simulink model "Copter_System_discrete"  (Simulink 7.4)
settings: Solver=ode4  StartTime=0.0  StopTime=tend  FixedStep=Ts  RelTol=1e-3
values from neighbouring files (symbols this model uses):
  dis_thrust = round(thrust.*shift)    [quadrocopter_param.m]
  f1 = (I_y-I_z)/I_x    [quadrocopter_param.m]
  f2 = rot.J_z/I_x    [quadrocopter_param.m]
  f3 = (I_z-I_x)/I_y    [quadrocopter_param.m]
  f4 = rot.J_z/I_y    [quadrocopter_param.m]
  g = 9.81    [complementary_filter_param.m]    (also in quadrocopter_param.m)
  HPF = 0.95    [complementary_filter_param.m]    (also in quadrocopter_param.m)
  I_x = elec.I_x+bat.I_x+2*boom.I_1x+2*boom.I_1y+2*mot.I_1x+2*mot.I_1y+                             2*rot.I_1x+2*rot.I_1y    [quadrocopter_param.m]
  I_y = elec.I_y+bat.I_y+2*boom.I_1x+2*boom.I_1y+2*mot.I_1x+2*mot.I_1y+                             2*rot.I_1x+2*rot.I_1y    [quadrocopter_param.m]
  I_z = elec.I_z+bat.I_z+4*boom.I_1z+4*mot.I_1z+4*rot.I_1z    [quadrocopter_param.m]
  LPF = 0.05    [complementary_filter_param.m]    (also in quadrocopter_param.m)
  m = elec.m+bat.m+boom.m+(4*mot.m)+(4*rot.m)    [quadrocopter_param.m]
  rpm = [1988 2544 2940 3566 4033 4500 5033 5233]    [quadrocopter_param.m]
  shift = 1000    [quadrocopter_param.m]
  speed = rpm.*(2*pi/60)    [quadrocopter_param.m]
  thrust = [0.58 1 1.33 2 2.54 3.33 4.08 4.54]    [quadrocopter_param.m]
  Ts = 0.01    [complementary_filter_param.m]    (also in quadrocopter_param.m)
undefined symbols (not defined in the file or in its folder): boom, DiscIntNeverNeededParam
libraries: simulink x11, dspinverses x1
settings Model: Creator=Joachim  LastModifiedBy=Sreekanth
settings DataIOCC: LimitDataPoints=off  SaveOutput=off  SaveState=on

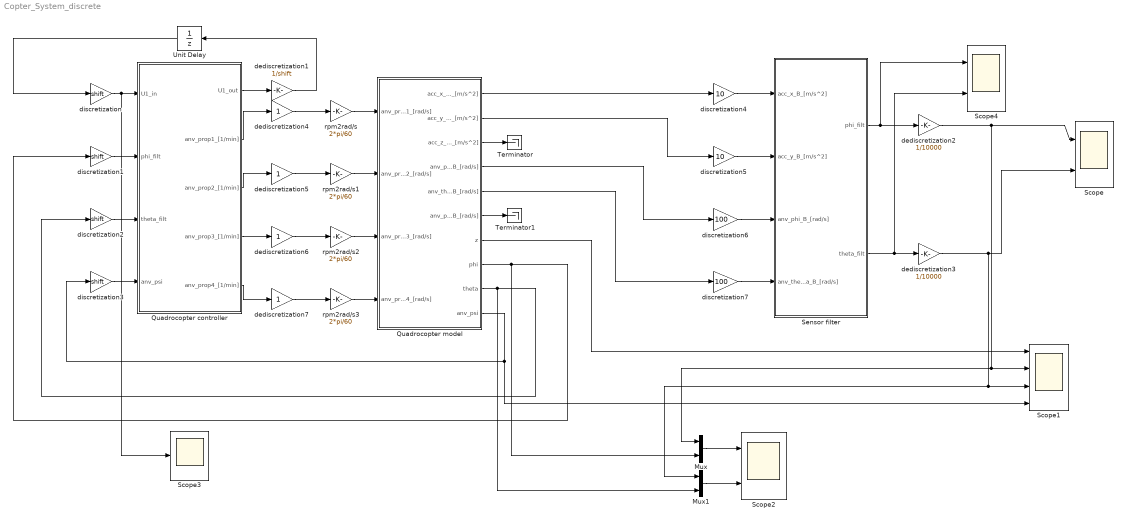
== system Copter_System_discrete ==
  Mux : Mux  Inputs=2
  Mux1 : Mux  Inputs=2
  Quadrocopter controller : Subsystem
  Quadrocopter model : Subsystem
  Scope : Scope  NumInputPorts=2
      settings: YMin=-5~-5  YMax=5~5  SaveName=ScopeData12
  Scope1 : Scope  NumInputPorts=4
      settings: YMin=-5~-5~-5~-5  YMax=5~5~5~5  SaveName=ScopeData14
  Scope2 : Scope  NumInputPorts=2
      settings: TimeRange=2.768662838392125  YMin=-0.00272445~-0.0178576  YMax=0.0152582~0.00343767  SaveName=ScopeData15
  Scope3 : Scope
      settings: TimeRange=2.768662838392125  YMin=-0.00272445  YMax=0.0152582  SaveName=ScopeData25
  Scope4 : Scope  NumInputPorts=2
      settings: YMin=-5~-5  YMax=5~5  SaveName=ScopeData27
  Sensor filter : Subsystem
  Terminator : Terminator
  Terminator1 : Terminator
  Unit Delay : UnitDelay  SampleTime=-1
  dediscretization1 : Gain  Gain=1/shift  ParameterDataType=fixdt(1, 16)  ParameterScaling=2^0  OutDataTypeMode=double  OutDataType=fixdt(1, 16)  OutScaling=2^0  OutDataTypeStr=double
  dediscretization2 : Gain  Gain=1/10000  ParameterDataType=fixdt(1, 16)  ParameterScaling=2^0  OutDataTypeMode=double  OutDataType=fixdt(1, 16)  OutScaling=2^0  OutDataTypeStr=double
  dediscretization3 : Gain  Gain=1/10000  ParameterDataType=fixdt(1, 16)  ParameterScaling=2^0  OutDataTypeMode=double  OutDataType=fixdt(1, 16)  OutScaling=2^0  OutDataTypeStr=double
  dediscretization{4..7} (4 alike) : Gain  ParameterDataType=fixdt(1, 16)  ParameterScaling=2^0  OutDataTypeMode=double  OutDataType=fixdt(1, 16)  OutScaling=2^0  OutDataTypeStr=double
  discretization{,1..3} (4 alike) : Gain  Gain=shift  ParameterDataType=fixdt(1, 16)  ParameterScaling=2^0  OutDataTypeMode=int16  OutDataType=fixdt(1, 16)  OutScaling=2^0  OutDataTypeStr=int16
  discretization4 : Gain  Gain=10  ParameterDataType=fixdt(1, 16)  ParameterScaling=2^0  OutDataTypeMode=int16  OutDataType=fixdt(1, 16)  OutScaling=2^0  OutDataTypeStr=int16
  discretization5 : Gain  Gain=10  ParameterDataType=fixdt(1, 16)  ParameterScaling=2^0  OutDataTypeMode=int16  OutDataType=fixdt(1, 16)  OutScaling=2^0  OutDataTypeStr=int16
  discretization6 : Gain  Gain=100  ParameterDataType=fixdt(1, 16)  ParameterScaling=2^0  OutDataTypeMode=int16  OutDataType=fixdt(1, 16)  OutScaling=2^0  OutDataTypeStr=int16
  discretization7 : Gain  Gain=100  ParameterDataType=fixdt(1, 16)  ParameterScaling=2^0  OutDataTypeMode=int16  OutDataType=fixdt(1, 16)  OutScaling=2^0  OutDataTypeStr=int16
  rpm2rad/s{,1..3} (4 alike) : Gain  Gain=2*pi/60  ParameterDataType=fixdt(1, 16)  ParameterScaling=2^0  OutDataType=fixdt(1, 16)  OutScaling=2^0
  wires:
  Quadrocopter controller/2(anv_prop1_[1/min]) -> dediscretization4/1
  Quadrocopter controller/3(anv_prop2_[1/min]) -> dediscretization5/1
  Quadrocopter controller/4(anv_prop3_[1/min]) -> dediscretization6/1
  Quadrocopter controller/5(anv_prop4_[1/min]) -> dediscretization7/1
  Quadrocopter model/7(z) -> Scope1/1
  Quadrocopter model/10(anv_psi) -> Scope1/4, discretization3/1
  Sensor filter/1(phi_filt) -> dediscretization2/1, Scope4/1
  Sensor filter/2(theta_filt) -> dediscretization3/1, Scope4/2
  Quadrocopter model/8(phi) -> Mux/2, discretization1/1
  Quadrocopter model/9(theta) -> Mux1/2, discretization2/1
  Mux/1 -> Scope2/1
  Mux1/1 -> Scope2/2
  Quadrocopter model/1(acc_x_B_[m/s^2]) -> discretization4/1
  Quadrocopter model/2(acc_y_B_[m/s^2]) -> discretization5/1
  Quadrocopter model/4(anv_phi_B_[rad/s]) -> discretization6/1
  Quadrocopter model/5(anv_theta_B_[rad/s]) -> discretization7/1
  Quadrocopter model/6(anv_psi_B_[rad/s]) -> Terminator1/1
  Quadrocopter model/3(acc_z_B_[m/s^2]) -> Terminator/1
  rpm2rad/s/1 -> Quadrocopter model/1(anv_prop1_[rad/s])
  rpm2rad/s1/1 -> Quadrocopter model/2(anv_prop2_[rad/s])
  rpm2rad/s2/1 -> Quadrocopter model/3(anv_prop3_[rad/s])
  rpm2rad/s3/1 -> Quadrocopter model/4(anv_prop4_[rad/s])
  discretization/1 -> Quadrocopter controller/1(U1_in), Scope3/1
  discretization1/1 -> Quadrocopter controller/2(phi_filt)
  discretization2/1 -> Quadrocopter controller/3(theta_filt)
  discretization3/1 -> Quadrocopter controller/4(anv_psi)
  dediscretization4/1 -> rpm2rad/s/1
  dediscretization5/1 -> rpm2rad/s1/1
  dediscretization6/1 -> rpm2rad/s2/1
  dediscretization7/1 -> rpm2rad/s3/1
  Quadrocopter controller/1(U1_out) -> dediscretization1/1
  dediscretization1/1 -> Unit Delay/1
  Unit Delay/1 -> discretization/1
  discretization4/1 -> Sensor filter/1(acc_x_B_[m/s^2])
  discretization5/1 -> Sensor filter/2(acc_y_B_[m/s^2])
  discretization6/1 -> Sensor filter/3(anv_phi_B_[rad/s])
  discretization7/1 -> Sensor filter/4(anv_theta_B_[rad/s])
  dediscretization2/1 -> Scope/1, Scope1/2, Mux/1
  dediscretization3/1 -> Scope/2, Scope1/3, Mux1/1

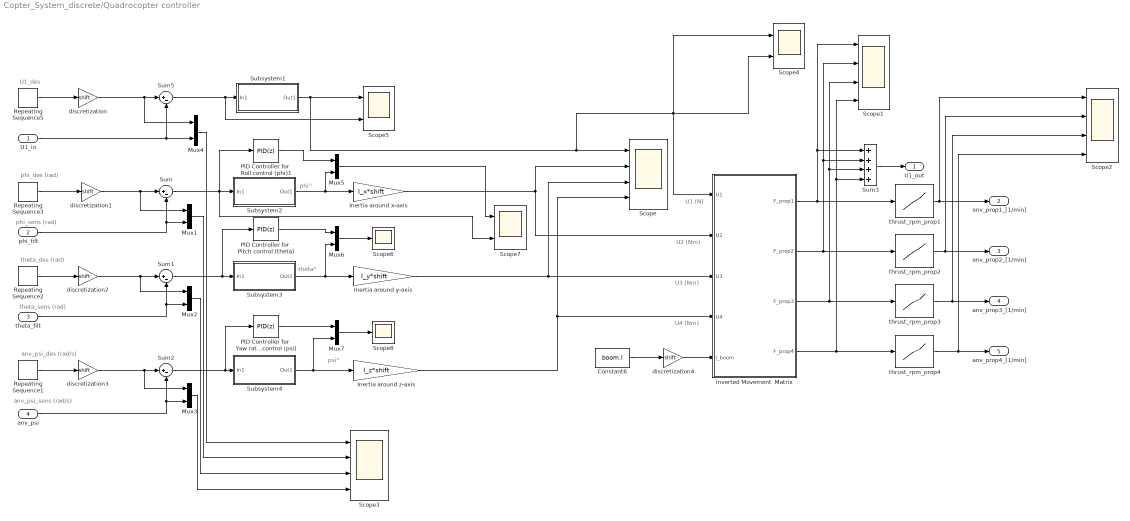
== system Copter_System_discrete/Quadrocopter controller ==
  note: U1 (N)
  note: U4 (Nm)
  note: U3 (Nm)
  note: U2 (Nm)
  note: anv_psi_sens (rad/s)
  note: anv_psi_des (rad/s)
  note: theta_sens (rad)
  note: theta_des (rad)
  note: phi_sens (rad)
  note: phi_des (rad)
  note: phi''
  note: theta''
  note: psi''
  note: U1_des
  U1_in : Inport  OutDataType=fixdt(1, 16)  OutScaling=2^0
  phi_filt : Inport  Port=2  OutDataType=fixdt(1, 16)  OutScaling=2^0
  theta_filt : Inport  Port=3  OutDataType=fixdt(1, 16)  OutScaling=2^0
  anv_psi : Inport  Port=4  OutDataType=fixdt(1, 16)  OutScaling=2^0
  Constant6 : Constant  Value=boom.l  OutDataType=fixdt(1, 16)  OutScaling=2^0  SampleTime=Ts
  Inertia around x-axis : Gain  Gain=I_x*shift  ParameterDataType=fixdt(1, 16)  ParameterScaling=2^0  OutDataType=fixdt(1, 16)  OutScaling=2^0  OutDataTypeStr=Inherit: Same as input
  Inertia around y-axis : Gain  Gain=I_y*shift  ParameterDataType=fixdt(1, 16)  ParameterScaling=2^0  OutDataType=fixdt(1, 16)  OutScaling=2^0  OutDataTypeStr=Inherit: Same as input
  Inertia around z-axis : Gain  Gain=I_z*shift  ParameterDataType=fixdt(1, 16)  ParameterScaling=2^0  OutDataType=fixdt(1, 16)  OutScaling=2^0  OutDataTypeStr=Inherit: Same as input
  Mux{1..7} (7 alike) : Mux  Inputs=2
  PID Controller for  Pitch control (theta) : simulink/Continuous/PID Controller  DialogController=pidpack.PIDConfig.pidDDGCreate  DialogControllerArgs=DataTag0  SystemSampleTime=-1  Controller=PID  TimeDomain=Discrete-time  SampleTime=Ts  IntegratorMethod=Forward Euler  FilterMethod=Forward Euler  Form=Parallel  P=20  I=5  D=10  N=100  InitialConditionSource=internal  InitialConditionForIntegrator=0  InitialConditionForFilter=0  ExternalReset=none  LimitOutput=off  UpperSaturationLimit=20  LowerSaturationLimit=-20  LinearizeAsGain=off  AntiWindupMode=clamping  Kb=1  TrackingMode=off  Kt=1  RndMeth=Nearest  PParamMin=[]  PParamMax=[]  PParamDataTypeStr=int16  IParamMin=[]  IParamMax=[]  IParamDataTypeStr=int16  DParamMin=[]  DParamMax=[]  DParamDataTypeStr=int16  NParamMin=[]  NParamMax=[]  NParamDataTypeStr=int16  KbParamMin=[]  KbParamMax=[]  KtParamMin=[]  KtParamMax=[]  POutMin=[]  POutMax=[]  POutDataTypeStr=int16  IOutMin=[]  IOutMax=[]  IOutDataTypeStr=int16  DOutMin=[]  DOutMax=[]  DOutDataTypeStr=int16  NOutMin=[]  NOutMax=[]  NOutDataTypeStr=int16  KbOutMin=[]  KbOutMax=[]  KtOutMin=[]  KtOutMax=[]  IntegratorOutMin=[]  IntegratorOutMax=[]  IntegratorOutDataTypeStr=int16  FilterOutMin=[]  FilterOutMax=[]  FilterOutDataTypeStr=int16  SumOutMin=[]  SumOutMax=[]  SumOutDataTypeStr=int16  SumI1OutMin=[]  SumI1OutMax=[]  SumI2OutMin=[]  SumI2OutMax=[]  SumI3OutMin=[]  SumI3OutMax=[]  SumDOutMin=[]  SumDOutMax=[]  SumDOutDataTypeStr=int16  SumAccumDataTypeStr=int16  SumDAccumDataTypeStr=int16  SaturationOutMin=[]  SaturationOutMax=[]  IntegratorContinuousStateAttributes=''  IntegratorStateMustResolveToSignalObject=off  IntegratorRTWStateStorageClass=Auto  FilterContinuousStateAttributes=''  FilterStateMustResolveToSignalObject=off  FilterRTWStateStorageClass=Auto
  PID Controller for  Roll control (phi)1 : simulink/Continuous/PID Controller  DialogController=pidpack.PIDConfig.pidDDGCreate  DialogControllerArgs=DataTag1  SystemSampleTime=-1  Controller=PID  TimeDomain=Discrete-time  SampleTime=Ts  IntegratorMethod=Forward Euler  FilterMethod=Forward Euler  Form=Parallel  P=20  I=5  D=1  N=150  InitialConditionSource=internal  InitialConditionForIntegrator=0  InitialConditionForFilter=0  ExternalReset=none  LimitOutput=off  UpperSaturationLimit=20  LowerSaturationLimit=-20  LinearizeAsGain=off  AntiWindupMode=clamping  Kb=1  TrackingMode=off  Kt=1  RndMeth=Nearest  PParamMin=[]  PParamMax=[]  PParamDataTypeStr=int16  IParamMin=[]  IParamMax=[]  IParamDataTypeStr=int16  DParamMin=[]  DParamMax=[]  DParamDataTypeStr=int16  NParamMin=[]  NParamMax=[]  NParamDataTypeStr=int16  KbParamMin=[]  KbParamMax=[]  KtParamMin=[]  KtParamMax=[]  POutMin=[]  POutMax=[]  POutDataTypeStr=int16  IOutMin=[]  IOutMax=[]  IOutDataTypeStr=int16  DOutMin=[]  DOutMax=[]  DOutDataTypeStr=int16  NOutMin=[]  NOutMax=[]  NOutDataTypeStr=int16  KbOutMin=[]  KbOutMax=[]  KtOutMin=[]  KtOutMax=[]  IntegratorOutMin=[]  IntegratorOutMax=[]  IntegratorOutDataTypeStr=int16  FilterOutMin=[]  FilterOutMax=[]  FilterOutDataTypeStr=int16  SumOutMin=[]  SumOutMax=[]  SumOutDataTypeStr=int16  SumI1OutMin=[]  SumI1OutMax=[]  SumI2OutMin=[]  SumI2OutMax=[]  SumI3OutMin=[]  SumI3OutMax=[]  SumDOutMin=[]  SumDOutMax=[]  SumDOutDataTypeStr=int16  SumAccumDataTypeStr=int16  SumDAccumDataTypeStr=int16  SaturationOutMin=[]  SaturationOutMax=[]  IntegratorContinuousStateAttributes=''  IntegratorStateMustResolveToSignalObject=off  IntegratorRTWStateStorageClass=Auto  FilterContinuousStateAttributes=''  FilterStateMustResolveToSignalObject=off  FilterRTWStateStorageClass=Auto
  PID Controller for  Yaw rate control (psi) : simulink/Continuous/PID Controller  DialogController=pidpack.PIDConfig.pidDDGCreate  DialogControllerArgs=DataTag2  SystemSampleTime=-1  Controller=PID  TimeDomain=Discrete-time  SampleTime=Ts  IntegratorMethod=Forward Euler  FilterMethod=Forward Euler  Form=Parallel  P=20.668455527077  I=1.53437531872718  D=9.7077013229996  N=3.52327682270198  InitialConditionSource=internal  InitialConditionForIntegrator=0  InitialConditionForFilter=0  ExternalReset=none  LimitOutput=off  UpperSaturationLimit=180  LowerSaturationLimit=-180  LinearizeAsGain=off  AntiWindupMode=clamping  Kb=1  TrackingMode=off  Kt=1  RndMeth=Nearest  PParamMin=[]  PParamMax=[]  PParamDataTypeStr=int16  IParamMin=[]  IParamMax=[]  IParamDataTypeStr=int16  DParamMin=[]  DParamMax=[]  DParamDataTypeStr=int16  NParamMin=[]  NParamMax=[]  NParamDataTypeStr=int16  KbParamMin=[]  KbParamMax=[]  KtParamMin=[]  KtParamMax=[]  POutMin=[]  POutMax=[]  POutDataTypeStr=int16  IOutMin=[]  IOutMax=[]  IOutDataTypeStr=int16  DOutMin=[]  DOutMax=[]  DOutDataTypeStr=int16  NOutMin=[]  NOutMax=[]  NOutDataTypeStr=int16  KbOutMin=[]  KbOutMax=[]  KtOutMin=[]  KtOutMax=[]  IntegratorOutMin=[]  IntegratorOutMax=[]  IntegratorOutDataTypeStr=int16  FilterOutMin=[]  FilterOutMax=[]  FilterOutDataTypeStr=int16  SumOutMin=[]  SumOutMax=[]  SumOutDataTypeStr=int16  SumI1OutMin=[]  SumI1OutMax=[]  SumI2OutMin=[]  SumI2OutMax=[]  SumI3OutMin=[]  SumI3OutMax=[]  SumDOutMin=[]  SumDOutMax=[]  SumDOutDataTypeStr=int16  SumAccumDataTypeStr=int16  SumDAccumDataTypeStr=int16  SaturationOutMin=[]  SaturationOutMax=[]  IntegratorContinuousStateAttributes=''  IntegratorStateMustResolveToSignalObject=off  IntegratorRTWStateStorageClass=Auto  FilterContinuousStateAttributes=''  FilterStateMustResolveToSignalObject=off  FilterRTWStateStorageClass=Auto
  Repeating Sequence1 : simulink/Sources/Repeating Sequence  SystemSampleTime=-1  rep_seq_t=desyaw.time  rep_seq_y=desyaw.velocity
  Repeating Sequence2 : simulink/Sources/Repeating Sequence  SystemSampleTime=-1  rep_seq_t=despitch.time  rep_seq_y=despitch.angle
  Repeating Sequence3 : simulink/Sources/Repeating Sequence  SystemSampleTime=-1  rep_seq_t=desroll.time  rep_seq_y=desroll.angle
  Repeating Sequence5 : simulink/Sources/Repeating Sequence  SystemSampleTime=-1  rep_seq_t=desforce.time  rep_seq_y=desforce.force
  Scope{,1..3} (4 alike) : Scope  NumInputPorts=4
      Scope settings: TimeRange=30  YMin=0~-2000~-20000~-1000  YMax=8000~2000~20000~1000
      Scope1 settings: TimeRange=30  YMin=-5~-5~-5~-5  YMax=5~5~5~5
      Scope2 settings: TimeRange=10  YMin=0~0~0~0  YMax=10000~10000~10000~10000  SaveName=ScopeData2
      Scope3 settings: TimeRange=10  YMin=-1e-015~0.359533~0.366931~0.234953  YMax=1e-015~0.397379~0.366932~0.259685  SaveName=ScopeData13
  Scope4 : Scope  NumInputPorts=2
      settings: TimeRange=30  YMin=0~0  YMax=10~10  SaveName=ScopeData21
  Scope5 : Scope  NumInputPorts=2
      settings: TimeRange=0.07528461379538221  YMin=832.2002173650526~0  YMax=840.8948194662481~900  SaveName=ScopeData23
  Scope6 : Scope
      settings: TimeRange=30  YMin=0  YMax=10  SaveName=ScopeData24
  Scope7 : Scope  NumInputPorts=2
      settings: TimeRange=30  YMin=0~0  YMax=10~10  SaveName=ScopeData26
  Scope8 : Scope
      settings: TimeRange=30  YMin=0  YMax=10  SaveName=ScopeData29
  Subsystem1 : Subsystem
  Subsystem2 : Subsystem
  Subsystem3 : Subsystem
  Subsystem4 : Subsystem
  Sum{,1..2,5} (4 alike) : Sum  Inputs=|+-  OutDataType=fixdt(1, 16)  OutScaling=2^0
  Sum3 : Sum  Inputs=++++  OutDataType=fixdt(1, 16)  OutScaling=2^0
  discretization{,1..4} (5 alike) : Gain  Gain=shift  ParameterDataType=fixdt(1, 16)  ParameterScaling=2^0  OutDataTypeMode=int16  OutDataType=fixdt(1, 16)  OutScaling=2^0  OutDataTypeStr=int16
  inverted Movement  Matrix : Stateflow chart
  thrust_rpm_prop{1..4} (4 alike) : Lookup  InputValues=dis_thrust  Table=rpm  LookUpMeth=Interpolation-Use End Values  OutDataType=fixdt(1, 16)  OutScaling=2^0
  U1_out : Outport  OutDataType=fixdt(1, 16)  OutScaling=2^0
  anv_prop1_[1/min] : Outport  Port=2  OutDataType=fixdt(1, 16)  OutScaling=2^0
  anv_prop2_[1/min] : Outport  Port=3  OutDataType=fixdt(1, 16)  OutScaling=2^0
  anv_prop3_[1/min] : Outport  Port=4  OutDataType=fixdt(1, 16)  OutScaling=2^0
  anv_prop4_[1/min] : Outport  Port=5  OutDataType=fixdt(1, 16)  OutScaling=2^0
  wires:
  Repeating Sequence1/1 -> discretization3/1
  Repeating Sequence2/1 -> discretization2/1
  Repeating Sequence3/1 -> discretization1/1
  theta_filt/1 -> Sum1/2, Mux2/2
  anv_psi/1 -> Sum2/2, Mux3/2
  phi_filt/1 -> Sum/2, Mux1/2
  thrust_rpm_prop2/1 -> anv_prop2_[1/min]/1, Scope2/2
  inverted Movement  Matrix/4(F_prop4) -> thrust_rpm_prop4/1, Scope1/4, Sum3/4
  inverted Movement  Matrix/3(F_prop3) -> thrust_rpm_prop3/1, Scope1/3, Sum3/3
  inverted Movement  Matrix/2(F_prop2) -> thrust_rpm_prop2/1, Scope1/2, Sum3/2
  inverted Movement  Matrix/1(F_prop1) -> thrust_rpm_prop1/1, Scope1/1, Sum3/1
  Inertia around x-axis/1 -> inverted Movement  Matrix/2(U2), Scope/2
  thrust_rpm_prop4/1 -> anv_prop4_[1/min]/1, Scope2/4
  thrust_rpm_prop3/1 -> anv_prop3_[1/min]/1, Scope2/3
  thrust_rpm_prop1/1 -> anv_prop1_[1/min]/1, Scope2/1
  Constant6/1 -> discretization4/1
  Inertia around z-axis/1 -> inverted Movement  Matrix/4(U4), Scope/4
  Inertia around y-axis/1 -> inverted Movement  Matrix/3(U3), Scope/3
  Sum2/1 -> PID Controller for  Yaw rate control (psi)/1, Subsystem4/1(In1)
  Sum1/1 -> PID Controller for  Pitch control (theta)/1, Subsystem3/1(In1)
  Sum/1 -> Subsystem2/1(In1), PID Controller for  Roll control (phi)1/1, Scope7/2
  Mux1/1 -> Scope3/2
  Mux2/1 -> Scope3/3
  Mux3/1 -> Scope3/4
  Repeating Sequence5/1 -> discretization/1
  Sum5/1 -> Subsystem1/1(In1), Scope5/2
  U1_in/1 -> Sum5/2, Mux4/2
  Mux4/1 -> Scope3/1
  discretization/1 -> Sum5/1, Mux4/1
  discretization1/1 -> Sum/1, Mux1/1
  discretization2/1 -> Sum1/1, Mux2/1
  discretization3/1 -> Sum2/1, Mux3/1
  discretization4/1 -> inverted Movement  Matrix/5(l_boom)
  Sum3/1 -> U1_out/1
  Subsystem1/1(Out1) -> inverted Movement  Matrix/1(U1), Scope4/1, Scope4/2, Scope/1, Scope5/1
  PID Controller for  Roll control (phi)1/1 -> Mux5/1
  Mux5/1 -> Scope7/1
  Subsystem2/1(Out1) -> Mux5/2, Inertia around x-axis/1
  Subsystem3/1(Out1) -> Inertia around y-axis/1, Mux6/2
  Mux6/1 -> Scope6/1
  PID Controller for  Pitch control (theta)/1 -> Mux6/1
  Subsystem4/1(Out1) -> Inertia around z-axis/1, Mux7/2
  Mux7/1 -> Scope8/1
  PID Controller for  Yaw rate control (psi)/1 -> Mux7/1

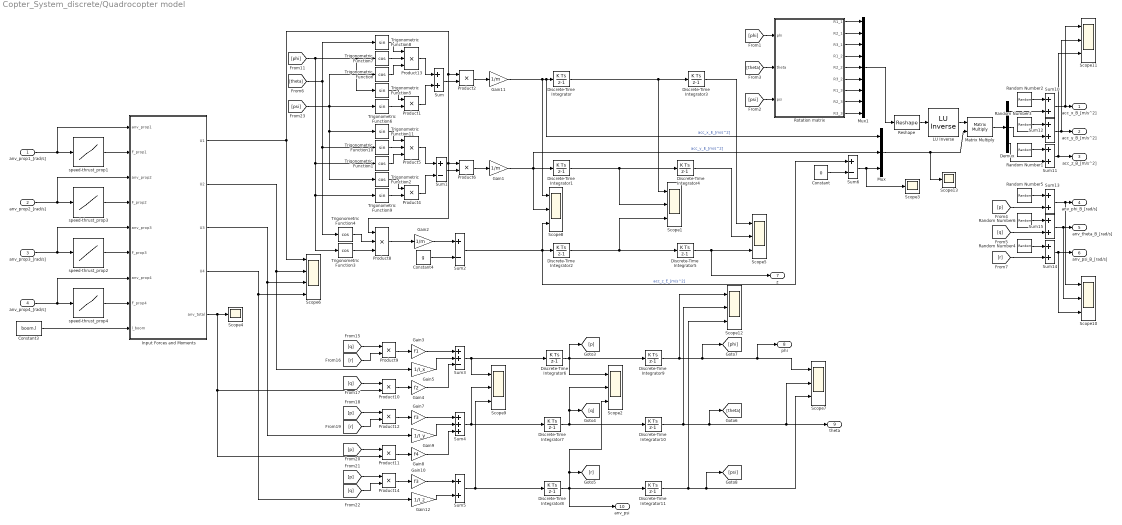
== system Copter_System_discrete/Quadrocopter model ==
  anv_prop1_[rad/s] : Inport  OutDataType=fixdt(1, 16)  OutScaling=2^0
  anv_prop2_[rad/s] : Inport  Port=2  OutDataType=fixdt(1, 16)  OutScaling=2^0
  anv_prop3_[rad/s] : Inport  Port=3  OutDataType=fixdt(1, 16)  OutScaling=2^0
  anv_prop4_[rad/s] : Inport  Port=4  OutDataType=fixdt(1, 16)  OutScaling=2^0
  " LU Inverse" : dspinverses/ LU Inverse  SystemSampleTime=-1
  Constant : Constant  Value=0  OutDataType=fixdt(1, 16)  OutScaling=2^0  SampleTime=Ts
  Constant3 : Constant  Value=boom.l  OutDataType=fixdt(1, 16)  OutScaling=2^0
  Constant4 : Constant  Value=g  OutDataType=fixdt(1, 16)  OutScaling=2^0  SampleTime=Ts
  Demux : Demux  Outputs=3
  Discrete-Time Integrator{,1..11} (12 alike) : DiscreteIntegrator  SampleTime=Ts  OutDataType=fixdt(1, 16)  OutScaling=2^0  ICPrevOutput=DiscIntNeverNeededParam  ICPrevScaledInput=DiscIntNeverNeededParam
  Gain1 : Gain  Gain=1/m  ParameterDataType=fixdt(1, 16)  ParameterScaling=2^0  OutDataType=fixdt(1, 16)  OutScaling=2^0
  Gain10 : Gain  Gain=f3  ParameterDataType=fixdt(1, 16)  ParameterScaling=2^0  OutDataType=fixdt(1, 16)  OutScaling=2^0
  Gain11 : Gain  Gain=1/m  ParameterDataType=fixdt(1, 16)  ParameterScaling=2^0  OutDataType=fixdt(1, 16)  OutScaling=2^0
  Gain12 : Gain  Gain=1/I_z  ParameterDataType=fixdt(1, 16)  ParameterScaling=2^0  OutDataType=fixdt(1, 16)  OutScaling=2^0
  Gain2 : Gain  Gain=1/m  ParameterDataType=fixdt(1, 16)  ParameterScaling=2^0  OutDataType=fixdt(1, 16)  OutScaling=2^0
  Gain3 : Gain  Gain=f1  ParameterDataType=fixdt(1, 16)  ParameterScaling=2^0  OutDataType=fixdt(1, 16)  OutScaling=2^0
  Gain4 : Gain  Gain=f2  ParameterDataType=fixdt(1, 16)  ParameterScaling=2^0  OutDataType=fixdt(1, 16)  OutScaling=2^0
  Gain5 : Gain  Gain=1/I_x  ParameterDataType=fixdt(1, 16)  ParameterScaling=2^0  OutDataType=fixdt(1, 16)  OutScaling=2^0
  Gain7 : Gain  Gain=f3  ParameterDataType=fixdt(1, 16)  ParameterScaling=2^0  OutDataType=fixdt(1, 16)  OutScaling=2^0
  Gain8 : Gain  Gain=f4  ParameterDataType=fixdt(1, 16)  ParameterScaling=2^0  OutDataType=fixdt(1, 16)  OutScaling=2^0
  Gain9 : Gain  Gain=1/I_y  ParameterDataType=fixdt(1, 16)  ParameterScaling=2^0  OutDataType=fixdt(1, 16)  OutScaling=2^0
  Input Forces and Moments : Stateflow chart
  Matrix Multiply : Product  Multiplication=Matrix(*)  OutDataType=sfix(16)  OutScaling=2^0
  Mux : Mux  Inputs=3
  Mux1 : Mux  Inputs=9
  Product{1..2,4,6,9..12,14} (9 alike) : Product  OutDataType=fixdt(1, 16)  OutScaling=2^0  RndMeth=Zero
  Product13 : Product  Inputs=3  OutDataType=fixdt(1, 16)  OutScaling=2^0  RndMeth=Zero
  Product5 : Product  Inputs=3  OutDataType=fixdt(1, 16)  OutScaling=2^0  RndMeth=Zero
  Product8 : Product  Inputs=3  OutDataType=fixdt(1, 16)  OutScaling=2^0  RndMeth=Zero
  Random Number{1..6} (6 alike) : RandomNumber  Variance=0  SampleTime=Ts
  Reshape : Reshape  OutputDimensionality=Customize  OutputDimensions=[3,3]
  Rotation matrix : Stateflow chart
  Scope{1..2,5,7..12} (9 alike) : Scope  NumInputPorts=3
      Scope1 settings: YMin=-5~-5~-5  YMax=5~5~5
      Scope10 settings: YMin=-5~-5~-5  YMax=5~5~5  SaveName=ScopeData9
      Scope11 settings: YMin=-5~-5~-5  YMax=5~5~5  SaveName=ScopeData10
      Scope12 settings: YMin=-5~-5~-5  YMax=5~5~5  SaveName=ScopeData11
      Scope2 settings: YMin=-5~-5~-5  YMax=5~5~5
      Scope5 settings: YMin=-5~-5~-5  YMax=5~5~5  SaveName=ScopeData3
      Scope7 settings: TimeRange=30  YMin=-0.05~-0.2~-0.5  YMax=0.3~0.15~3  SaveName=ScopeData6
      Scope8 settings: TimeRange=30  YMin=-1~-1~3  YMax=1~1~10  SaveName=ScopeData7
      Scope9 settings: YMin=-5~-5~-5  YMax=5~5~5  SaveName=ScopeData8
  Scope13 : Scope
      settings: SaveName=ScopeData22
  Scope3 : Scope
      settings: SaveName=ScopeData19
  Scope4 : Scope
      settings: SaveName=ScopeData4
  Scope6 : Scope  NumInputPorts=4
      settings: YMin=-5~-5~-5~-5  YMax=5~5~5~5  SaveName=ScopeData5
  Sum{,5,10..15} (8 alike) : Sum  OutDataType=fixdt(1, 16)  OutScaling=2^0
  Sum1 : Sum  Inputs=+-  OutDataType=fixdt(1, 16)  OutScaling=2^0
  Sum2 : Sum  Inputs=+-  OutDataType=fixdt(1, 16)  OutScaling=2^0
  Sum3 : Sum  Inputs=++-  OutDataType=fixdt(1, 16)  OutScaling=2^0
  Sum4 : Sum  Inputs=+++  OutDataType=fixdt(1, 16)  OutScaling=2^0
  Sum6 : Sum  Inputs=+-  OutDataType=fixdt(1, 16)  OutScaling=2^0
  Trigonometric Function{,1..4,7} (6 alike) : Trigonometry  Operator=cos
  Trigonometric Function{5..6,8..11} (6 alike) : Trigonometry
  speed-thrust_prop{1..4} (4 alike) : Lookup  InputValues=speed  Table=thrust  LookUpMeth=Interpolation-Use End Values  OutDataType=fixdt(1, 16)  OutScaling=2^0
  acc_x_B_[m/s^2] : Outport  OutDataType=fixdt(1, 16)  OutScaling=2^0
  acc_y_B_[m/s^2] : Outport  Port=2  OutDataType=fixdt(1, 16)  OutScaling=2^0
  acc_z_B_[m/s^2] : Outport  Port=3  OutDataType=fixdt(1, 16)  OutScaling=2^0
  anv_phi_B_[rad/s] : Outport  Port=4  OutDataType=fixdt(1, 16)  OutScaling=2^0
  anv_theta_B_[rad/s] : Outport  Port=5  OutDataType=fixdt(1, 16)  OutScaling=2^0
  anv_psi_B_[rad/s] : Outport  Port=6  OutDataType=fixdt(1, 16)  OutScaling=2^0
  z : Outport  Port=7  OutDataType=fixdt(1, 16)  OutScaling=2^0
  phi : Outport  Port=8  OutDataType=fixdt(1, 16)  OutScaling=2^0
  theta : Outport  Port=9  OutDataType=fixdt(1, 16)  OutScaling=2^0
  anv_psi : Outport  Port=10  OutDataType=fixdt(1, 16)  OutScaling=2^0
  wires:
  Sum14/1 -> Scope10/3, anv_psi_B_[rad/s]/1
  Sum15/1 -> Scope10/2, anv_theta_B_[rad/s]/1
  Sum13/1 -> Scope10/1, anv_phi_B_[rad/s]/1
  [q] -> Sum15/2
  Random Number6/1 -> Sum15/1
  [r] -> Sum14/2
  Random Number4/1 -> Sum14/1
  [p] -> Sum13/2
  Random Number5/1 -> Sum13/1
  Sum11/1 -> Scope11/3, acc_z_B_[m/s^2]/1
  Sum12/1 -> Scope11/2, acc_y_B_[m/s^2]/1
  Sum10/1 -> Scope11/1, acc_x_B_[m/s^2]/1
  Demux/2 -> Sum12/2
  Random Number3/1 -> Sum12/1
  Demux/3 -> Sum11/2
  Random Number1/1 -> Sum11/1
  Demux/1 -> Sum10/2
  Random Number2/1 -> Sum10/1
  Matrix Multiply/1 -> Demux/1
  anv_prop3_[rad/s]/1 -> speed-thrust_prop2/1, Input Forces and Moments/5(anv_prop3)
  anv_prop4_[rad/s]/1 -> speed-thrust_prop4/1, Input Forces and Moments/7(anv_prop4)
  Reshape/1 -> " LU Inverse"/1
  Mux/1 -> Matrix Multiply/2, Scope13/1
  Mux1/1 -> Reshape/1
  Rotation matrix/9(R3_3) -> Mux1/9
  Rotation matrix/8(R2_3) -> Mux1/8
  Rotation matrix/7(R1_3) -> Mux1/7
  Rotation matrix/6(R3_2) -> Mux1/6
  Rotation matrix/5(R2_2) -> Mux1/5
  Rotation matrix/4(R1_2) -> Mux1/4
  Rotation matrix/3(R3_1) -> Mux1/3
  Rotation matrix/2(R2_1) -> Mux1/2
  Rotation matrix/1(R1_1) -> Mux1/1
  [psi] -> Rotation matrix/3(psi)
  [theta] -> Rotation matrix/2(theta)
  [phi] -> Rotation matrix/1(phi)
  anv_prop2_[rad/s]/1 -> speed-thrust_prop3/1, Input Forces and Moments/3(anv_prop2)
  anv_prop1_[rad/s]/1 -> speed-thrust_prop1/1, Input Forces and Moments/1(anv_prop1)
  Constant4/1 -> Sum2/2
  Trigonometric Function4/1 -> Product8/2
  Trigonometric Function3/1 -> Product8/3
  Gain2/1 -> Sum2/1
  Gain11/1 -> Scope8/1, Discrete-Time Integrator/1, Mux/1  "acc_x_E_[m/s^2]"
  Product6/1 -> Gain1/1
  Sum1/1 -> Product6/2
  Product5/1 -> Sum1/1
  Trigonometric Function1/1 -> Product5/3
  Trigonometric Function10/1 -> Product5/2
  Trigonometric Function11/1 -> Product5/1
  Product4/1 -> Sum1/2
  Trigonometric Function2/1 -> Product4/1
  Trigonometric Function9/1 -> Product4/2
  Product2/1 -> Gain11/1
  Sum/1 -> Product2/2
  Product13/1 -> Sum/1
  Trigonometric Function/1 -> Product13/3
  Trigonometric Function7/1 -> Product13/2
  Trigonometric Function8/1 -> Product13/1
  Product1/1 -> Sum/2
  Trigonometric Function5/1 -> Product1/1
  Trigonometric Function6/1 -> Product1/2
  [psi] -> Trigonometric Function2/1, Trigonometric Function11/1, Trigonometric Function/1, Trigonometric Function6/1
  Discrete-Time Integrator/1 -> Scope1/1, Discrete-Time Integrator3/1
  Discrete-Time Integrator1/1 -> Scope1/2, Discrete-Time Integrator4/1
  Discrete-Time Integrator2/1 -> Scope1/3, Discrete-Time Integrator5/1
  [theta] -> Trigonometric Function10/1, Trigonometric Function4/1, Trigonometric Function8/1
  Gain1/1 -> Scope8/2, Discrete-Time Integrator1/1, Mux/2  "acc_y_E_[m/s^2]"
  [phi] -> Trigonometric Function9/1, Trigonometric Function3/1, Trigonometric Function1/1, Trigonometric Function7/1, Trigonometric Function5/1
  Product8/1 -> Gain2/1
  Sum2/1 -> Scope8/3, Discrete-Time Integrator2/1, Sum6/1  "acc_z_E_[m/s^2]"
  Discrete-Time Integrator3/1 -> Scope5/1
  Discrete-Time Integrator4/1 -> Scope5/2
  Discrete-Time Integrator5/1 -> Scope5/3, z/1
  Constant3/1 -> Input Forces and Moments/9(l_boom)
  Sum5/1 -> Scope9/3, Discrete-Time Integrator8/1
  Input Forces and Moments/4(U4) -> Scope6/4, Gain12/1
  Gain12/1 -> Sum5/2
  Gain10/1 -> Sum5/1
  Product14/1 -> Gain10/1
  [q] -> Product14/2
  [p] -> Product14/1
  Sum4/1 -> Scope9/2, Discrete-Time Integrator7/1
  Input Forces and Moments/3(U3) -> Scope6/3, Gain9/1
  Gain8/1 -> Sum4/3
  Gain9/1 -> Sum4/2
  Product11/1 -> Gain8/1
  [p] -> Product11/1
  Gain7/1 -> Sum4/1
  Product12/1 -> Gain7/1
  [r] -> Product12/2
  [p] -> Product12/1
  Input Forces and Moments/1(U1) -> Product8/1, Product6/1, Product2/1, Scope6/1
  Sum3/1 -> Scope9/1, Discrete-Time Integrator6/1
  Gain4/1 -> Sum3/3
  Gain5/1 -> Sum3/2
  Input Forces and Moments/2(U2) -> Scope6/2, Gain5/1
  Product10/1 -> Gain4/1
  [q] -> Product10/1
  Gain3/1 -> Sum3/1
  Product9/1 -> Gain3/1
  [r] -> Product9/2
  [q] -> Product9/1
  Input Forces and Moments/5(anv_total) -> Product11/2, Product10/2, Scope4/1
  Discrete-Time Integrator9/1 -> Scope12/1, [phi], Scope7/1, phi/1
  Discrete-Time Integrator10/1 -> Scope12/2, [theta], Scope7/2, theta/1
  Discrete-Time Integrator11/1 -> Scope12/3, Scope7/3, [psi]
  Discrete-Time Integrator6/1 -> Scope2/1, [p], Discrete-Time Integrator9/1
  Discrete-Time Integrator7/1 -> Scope2/2, [q], Discrete-Time Integrator10/1
  Discrete-Time Integrator8/1 -> Scope2/3, [r], anv_psi/1, Discrete-Time Integrator11/1
  speed-thrust_prop4/1 -> Input Forces and Moments/8(F_prop4)
  speed-thrust_prop1/1 -> Input Forces and Moments/2(F_prop1)
  speed-thrust_prop3/1 -> Input Forces and Moments/4(F_prop2)
  speed-thrust_prop2/1 -> Input Forces and Moments/6(F_prop3)
  Constant/1 -> Sum6/2
  Sum6/1 -> Mux/3, Scope3/1
  " LU Inverse"/1 -> Matrix Multiply/1

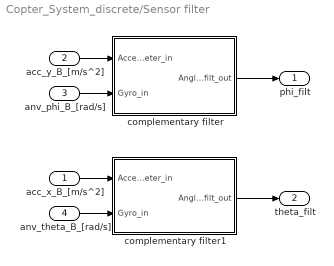
== system Copter_System_discrete/Sensor filter ==
  acc_x_B_[m/s^2] : Inport
  acc_y_B_[m/s^2] : Inport  Port=2
  anv_phi_B_[rad/s] : Inport  Port=3
  anv_theta_B_[rad/s] : Inport  Port=4
  complementary filter : Subsystem
  complementary filter1 : Subsystem
  phi_filt : Outport
  theta_filt : Outport  Port=2
  wires:
  complementary filter/1(Angle_filt_out) -> phi_filt/1
  anv_phi_B_[rad/s]/1 -> complementary filter/2(Gyro_in)
  complementary filter1/1(Angle_filt_out) -> theta_filt/1
  anv_theta_B_[rad/s]/1 -> complementary filter1/2(Gyro_in)
  acc_x_B_[m/s^2]/1 -> complementary filter1/1(Accelerometer_in)
  acc_y_B_[m/s^2]/1 -> complementary filter/1(Accelerometer_in)

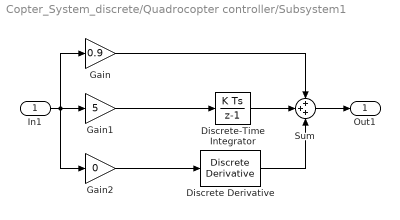
== system Copter_System_discrete/Quadrocopter controller/Subsystem1 ==
  In1 : Inport  OutDataType=fixdt(1, 16)  OutScaling=2^0
  Discrete Derivative : simulink/Discrete/Discrete Derivative  SystemSampleTime=-1  gainval=1.0  ICPrevScaledInput=0.0  OutMin=[]  OutMax=[]  OutDataTypeStr=int16  OutputDataTypeScalingMode=int16  OutDataType=fixdt(1, 16)  OutScaling=2^-10  DoSatur=off
  Discrete-Time Integrator : DiscreteIntegrator  SampleTime=Ts  OutDataTypeMode=int16  OutDataType=fixdt(1, 16)  OutScaling=2^0  OutDataTypeStr=int16  ICPrevOutput=DiscIntNeverNeededParam  ICPrevScaledInput=DiscIntNeverNeededParam
  Gain : Gain  Gain=0.9  ParameterDataType=fixdt(1, 16)  ParameterScaling=2^0  OutDataTypeMode=int16  OutDataType=fixdt(1, 16)  OutScaling=2^0  OutDataTypeStr=int16
  Gain1 : Gain  Gain=5  ParameterDataType=fixdt(1, 16)  ParameterScaling=2^0  OutDataTypeMode=int16  OutDataType=fixdt(1, 16)  OutScaling=2^0  OutDataTypeStr=int16
  Gain2 : Gain  Gain=0  ParameterDataType=fixdt(1, 16)  ParameterScaling=2^0  OutDataTypeMode=int16  OutDataType=fixdt(1, 16)  OutScaling=2^0  OutDataTypeStr=int16
  Sum : Sum  Inputs=+++  OutDataType=fixdt(1, 16)  OutScaling=2^0
  Out1 : Outport  OutDataType=fixdt(1, 16)  OutScaling=2^0
  wires:
  Sum/1 -> Out1/1
  Gain/1 -> Sum/1
  Discrete-Time Integrator/1 -> Sum/2
  Gain1/1 -> Discrete-Time Integrator/1
  Discrete Derivative/1 -> Sum/3
  Gain2/1 -> Discrete Derivative/1
  In1/1 -> Gain2/1, Gain/1, Gain1/1

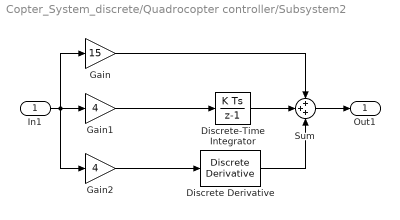
== system Copter_System_discrete/Quadrocopter controller/Subsystem2 ==
  In1 : Inport  OutDataType=fixdt(1, 16)  OutScaling=2^0
  Discrete Derivative : simulink/Discrete/Discrete Derivative  SystemSampleTime=-1  gainval=1.0  ICPrevScaledInput=0.0  OutMin=[]  OutMax=[]  OutDataTypeStr=int16  OutputDataTypeScalingMode=int16  OutDataType=fixdt(1, 16)  OutScaling=2^-10  DoSatur=off
  Discrete-Time Integrator : DiscreteIntegrator  SampleTime=Ts  OutDataTypeMode=int16  OutDataType=fixdt(1, 16)  OutScaling=2^0  OutDataTypeStr=int16  ICPrevOutput=DiscIntNeverNeededParam  ICPrevScaledInput=DiscIntNeverNeededParam
  Gain : Gain  Gain=15  ParameterDataType=fixdt(1, 16)  ParameterScaling=2^0  OutDataTypeMode=int16  OutDataType=fixdt(1, 16)  OutScaling=2^0  OutDataTypeStr=int16
  Gain1 : Gain  Gain=4  ParameterDataType=fixdt(1, 16)  ParameterScaling=2^0  OutDataTypeMode=int16  OutDataType=fixdt(1, 16)  OutScaling=2^0  OutDataTypeStr=int16
  Gain2 : Gain  Gain=4  ParameterDataType=fixdt(1, 16)  ParameterScaling=2^0  OutDataTypeMode=int16  OutDataType=fixdt(1, 16)  OutScaling=2^0  OutDataTypeStr=int16
  Sum : Sum  Inputs=+++  OutDataType=fixdt(1, 16)  OutScaling=2^0
  Out1 : Outport  OutDataType=fixdt(1, 16)  OutScaling=2^0
  wires:
  In1/1 -> Gain1/1, Gain/1, Gain2/1
  Gain2/1 -> Discrete Derivative/1
  Discrete Derivative/1 -> Sum/3
  Gain1/1 -> Discrete-Time Integrator/1
  Discrete-Time Integrator/1 -> Sum/2
  Gain/1 -> Sum/1
  Sum/1 -> Out1/1

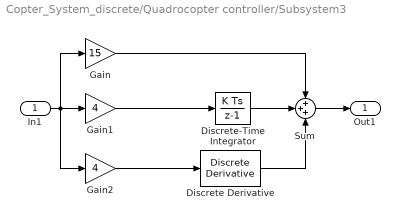
== system Copter_System_discrete/Quadrocopter controller/Subsystem3 ==
  In1 : Inport  OutDataType=fixdt(1, 16)  OutScaling=2^0
  Discrete Derivative : simulink/Discrete/Discrete Derivative  SystemSampleTime=-1  gainval=1.0  ICPrevScaledInput=0.0  OutMin=[]  OutMax=[]  OutDataTypeStr=int16  OutputDataTypeScalingMode=int16  OutDataType=fixdt(1, 16)  OutScaling=2^-10  DoSatur=off
  Discrete-Time Integrator : DiscreteIntegrator  SampleTime=Ts  OutDataTypeMode=int16  OutDataType=fixdt(1, 16)  OutScaling=2^0  OutDataTypeStr=int16  ICPrevOutput=DiscIntNeverNeededParam  ICPrevScaledInput=DiscIntNeverNeededParam
  Gain : Gain  Gain=15  ParameterDataType=fixdt(1, 16)  ParameterScaling=2^0  OutDataTypeMode=int16  OutDataType=fixdt(1, 16)  OutScaling=2^0  OutDataTypeStr=int16
  Gain1 : Gain  Gain=4  ParameterDataType=fixdt(1, 16)  ParameterScaling=2^0  OutDataTypeMode=int16  OutDataType=fixdt(1, 16)  OutScaling=2^0  OutDataTypeStr=int16
  Gain2 : Gain  Gain=4  ParameterDataType=fixdt(1, 16)  ParameterScaling=2^0  OutDataTypeMode=int16  OutDataType=fixdt(1, 16)  OutScaling=2^0  OutDataTypeStr=int16
  Sum : Sum  Inputs=+++  OutDataType=fixdt(1, 16)  OutScaling=2^0
  Out1 : Outport  OutDataType=fixdt(1, 16)  OutScaling=2^0
  wires:
  Sum/1 -> Out1/1
  Gain/1 -> Sum/1
  Discrete-Time Integrator/1 -> Sum/2
  Gain1/1 -> Discrete-Time Integrator/1
  Discrete Derivative/1 -> Sum/3
  Gain2/1 -> Discrete Derivative/1
  In1/1 -> Gain2/1, Gain/1, Gain1/1

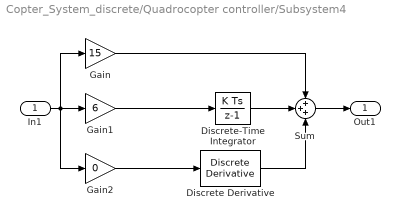
== system Copter_System_discrete/Quadrocopter controller/Subsystem4 ==
  In1 : Inport  OutDataType=fixdt(1, 16)  OutScaling=2^0
  Discrete Derivative : simulink/Discrete/Discrete Derivative  SystemSampleTime=-1  gainval=1.0  ICPrevScaledInput=0.0  OutMin=[]  OutMax=[]  OutDataTypeStr=int16  OutputDataTypeScalingMode=int16  OutDataType=fixdt(1, 16)  OutScaling=2^-10  DoSatur=off
  Discrete-Time Integrator : DiscreteIntegrator  SampleTime=Ts  OutDataTypeMode=int16  OutDataType=fixdt(1, 16)  OutScaling=2^0  OutDataTypeStr=int16  ICPrevOutput=DiscIntNeverNeededParam  ICPrevScaledInput=DiscIntNeverNeededParam
  Gain : Gain  Gain=15  ParameterDataType=fixdt(1, 16)  ParameterScaling=2^0  OutDataTypeMode=int16  OutDataType=fixdt(1, 16)  OutScaling=2^0  OutDataTypeStr=int16
  Gain1 : Gain  Gain=6  ParameterDataType=fixdt(1, 16)  ParameterScaling=2^0  OutDataTypeMode=int16  OutDataType=fixdt(1, 16)  OutScaling=2^0  OutDataTypeStr=int16
  Gain2 : Gain  Gain=0  ParameterDataType=fixdt(1, 16)  ParameterScaling=2^0  OutDataTypeMode=int16  OutDataType=fixdt(1, 16)  OutScaling=2^0  OutDataTypeStr=int16
  Sum : Sum  Inputs=+++  OutDataType=fixdt(1, 16)  OutScaling=2^0
  Out1 : Outport  OutDataType=fixdt(1, 16)  OutScaling=2^0
  wires:
  In1/1 -> Gain1/1, Gain/1, Gain2/1
  Gain2/1 -> Discrete Derivative/1
  Discrete Derivative/1 -> Sum/3
  Gain1/1 -> Discrete-Time Integrator/1
  Discrete-Time Integrator/1 -> Sum/2
  Gain/1 -> Sum/1
  Sum/1 -> Out1/1

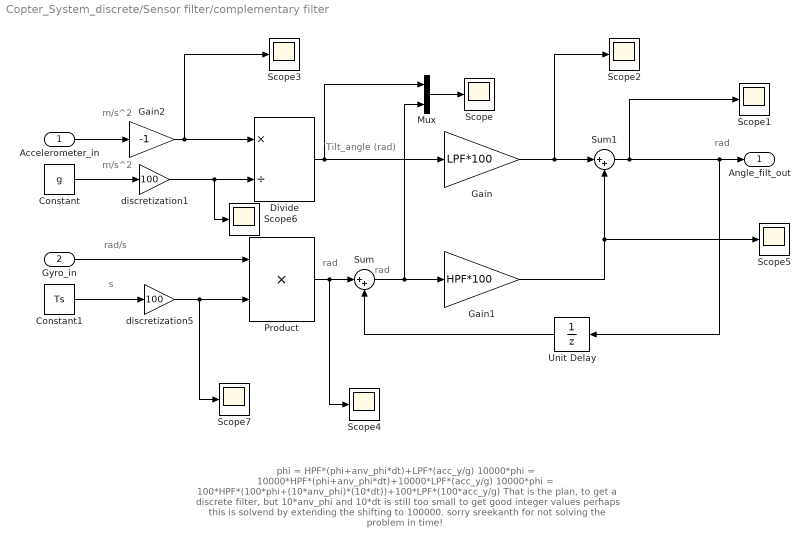
== system Copter_System_discrete/Sensor filter/complementary filter ==
  note: rad
  note: rad
  note: rad
  note: s
  note: rad/s
  note: m/s^2
  note: m/s^2
  note: Tilt_angle (rad)
  note: phi = HPF*(phi+anv_phi*dt)+LPF*(acc_y/g)
      | 10000*phi = 10000*HPF*(phi+anv_phi*dt)+10000*LPF*(acc_y/g)
      | 10000*phi = 100*HPF*(100*phi+(10*anv_phi)*(10*dt))+100*LPF*(100*acc_y/g)
      |
      | That is the plan, to get a discrete filter, but 10*anv_phi and 10*dt is still too small to get good integer values
      | perhaps this is solvend by extending the shifting to 100000. sorry sreekanth for not solving the problem in time!
  Accelerometer_in : Inport  OutDataType=fixdt(1, 16)  OutScaling=2^0
  Gyro_in : Inport  Port=2  OutDataType=fixdt(1, 16)  OutScaling=2^0
  Constant : Constant  Value=g  OutDataType=fixdt(1, 16)  OutScaling=2^0  SampleTime=Ts
  Constant1 : Constant  Value=Ts  OutDataType=fixdt(1, 16)  OutScaling=2^0  SampleTime=Ts
  Divide : Product  Inputs=*/  OutDataTypeMode=int16  OutDataType=fixdt(1, 16)  OutScaling=2^-10  OutDataTypeStr=int16
  Gain : Gain  Gain=LPF*100  ParameterDataType=fixdt(1, 16)  ParameterScaling=2^0  OutDataTypeMode=int16  OutDataType=fixdt(1, 16)  OutScaling=2^0  OutDataTypeStr=int16
  Gain1 : Gain  Gain=HPF*100  ParameterDataType=fixdt(1, 16)  ParameterScaling=2^0  OutDataTypeMode=int16  OutDataType=fixdt(1, 16)  OutScaling=2^0  OutDataTypeStr=int16
  Gain2 : Gain  Gain=-1  ParameterDataType=fixdt(1, 16)  ParameterScaling=2^0  OutDataTypeMode=int16  OutDataType=fixdt(1, 16)  OutScaling=2^0  OutDataTypeStr=int16
  Mux : Mux  Inputs=2
  Product : Product  OutDataTypeMode=int16  OutDataType=fixdt(1, 16)  OutScaling=2^0  OutDataTypeStr=int16  RndMeth=Nearest
  Scope{,1..7} (8 alike) : Scope
      Scope settings: SaveName=ScopeData16
      Scope1 settings: SaveName=ScopeData17
      Scope2 settings: SaveName=ScopeData20
      Scope3 settings: SaveName=ScopeData28
      Scope4 settings: SaveName=ScopeData30
      Scope5 settings: SaveName=ScopeData31
      Scope6 settings: SaveName=ScopeData32
      Scope7 settings: SaveName=ScopeData34
  Sum : Sum  Inputs=|++  OutDataTypeMode=int16  OutDataType=fixdt(1, 16)  OutScaling=2^0  OutDataTypeStr=int16
  Sum1 : Sum  Inputs=|++  OutDataTypeMode=int32  OutDataType=fixdt(1, 16)  OutScaling=2^0  OutDataTypeStr=int32
  Unit Delay : UnitDelay  SampleTime=-1
  discretization1 : Gain  Gain=100  ParameterDataType=fixdt(1, 16)  ParameterScaling=2^0  OutDataTypeMode=int16  OutDataType=fixdt(1, 16)  OutScaling=2^0  OutDataTypeStr=int16
  discretization5 : Gain  Gain=100  ParameterDataType=fixdt(1, 16)  ParameterScaling=2^0  OutDataTypeMode=int16  OutDataType=fixdt(1, 16)  OutScaling=2^0  OutDataTypeStr=int16
  Angle_filt_out : Outport  OutDataType=fixdt(1, 16)  OutScaling=2^0
  wires:
  Constant/1 -> discretization1/1
  Accelerometer_in/1 -> Gain2/1
  Gyro_in/1 -> Product/1
  Constant1/1 -> discretization5/1
  Sum/1 -> Gain1/1, Mux/2
  Sum1/1 -> Angle_filt_out/1, Unit Delay/1, Scope1/1
  Gain1/1 -> Scope5/1, Sum1/2
  Gain/1 -> Scope2/1, Sum1/1
  Product/1 -> Sum/1, Scope4/1
  Divide/1 -> Gain/1, Mux/1
  Mux/1 -> Scope/1
  Unit Delay/1 -> Sum/2
  Gain2/1 -> Scope3/1, Divide/1
  discretization5/1 -> Product/2, Scope7/1
  discretization1/1 -> Divide/2, Scope6/1

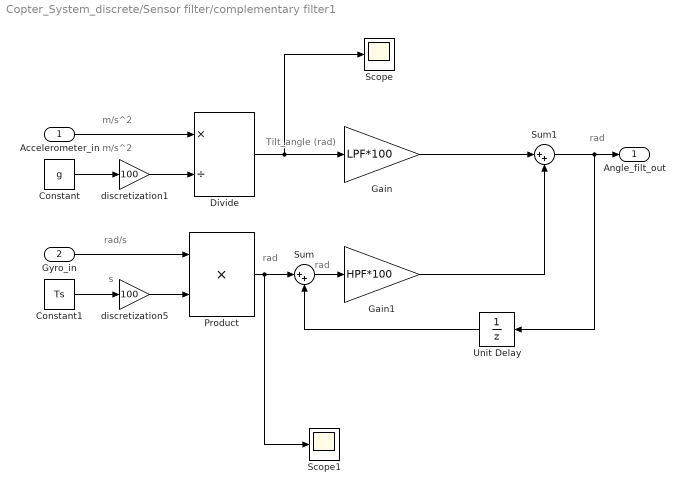
== system Copter_System_discrete/Sensor filter/complementary filter1 ==
  note: Tilt_angle (rad)
  note: m/s^2
  note: m/s^2
  note: rad/s
  note: s
  note: rad
  note: rad
  note: rad
  Accelerometer_in : Inport  OutDataType=fixdt(1, 16)  OutScaling=2^0
  Gyro_in : Inport  Port=2  OutDataType=fixdt(1, 16)  OutScaling=2^0
  Constant : Constant  Value=g  OutDataTypeMode=int16  OutDataType=fixdt(1, 16)  OutScaling=2^0  OutDataTypeStr=int16  SampleTime=Ts
  Constant1 : Constant  Value=Ts  OutDataType=fixdt(1, 16)  OutScaling=2^0  SampleTime=Ts
  Divide : Product  Inputs=*/  OutDataType=fixdt(1, 16)  OutScaling=2^-10
  Gain : Gain  Gain=LPF*100  ParameterDataType=fixdt(1, 16)  ParameterScaling=2^0  OutDataTypeMode=int16  OutDataType=fixdt(1, 16)  OutScaling=2^0  OutDataTypeStr=int16
  Gain1 : Gain  Gain=HPF*100  ParameterDataType=fixdt(1, 16)  ParameterScaling=2^0  OutDataTypeMode=int16  OutDataType=fixdt(1, 16)  OutScaling=2^0  OutDataTypeStr=int16
  Product : Product  OutDataType=fixdt(1, 16)  OutScaling=2^0  RndMeth=Zero
  Scope : Scope
      settings: SaveName=ScopeData18
  Scope1 : Scope
      settings: SaveName=ScopeData33
  Sum : Sum  Inputs=|++  OutDataType=fixdt(1, 16)  OutScaling=2^0
  Sum1 : Sum  Inputs=|++  AccumDataTypeStr=int16  OutDataType=fixdt(1, 16)  OutScaling=2^0
  Unit Delay : UnitDelay  SampleTime=-1
  discretization1 : Gain  Gain=100  ParameterDataType=fixdt(1, 16)  ParameterScaling=2^0  OutDataTypeMode=int16  OutDataType=fixdt(1, 16)  OutScaling=2^0  OutDataTypeStr=int16
  discretization5 : Gain  Gain=100  ParameterDataType=fixdt(1, 16)  ParameterScaling=2^0  OutDataTypeMode=int16  OutDataType=fixdt(1, 16)  OutScaling=2^0  OutDataTypeStr=int16
  Angle_filt_out : Outport  OutDataType=fixdt(1, 16)  OutScaling=2^0
  wires:
  Divide/1 -> Gain/1, Scope/1
  Product/1 -> Sum/1, Scope1/1
  Gain/1 -> Sum1/1
  Gain1/1 -> Sum1/2
  Sum1/1 -> Angle_filt_out/1, Unit Delay/1
  Sum/1 -> Gain1/1
  Constant1/1 -> discretization5/1
  Gyro_in/1 -> Product/1
  Accelerometer_in/1 -> Divide/1
  Constant/1 -> discretization1/1
  Unit Delay/1 -> Sum/2
  discretization5/1 -> Product/2
  discretization1/1 -> Divide/2

== matlab function Quadrocopter model/Input Forces and Moments ==
  data: anv_prop1 input double; F_prop1 input double; anv_prop2 input double; F_prop2 input double; anv_prop3 input double; F_prop3 input double; anv_prop4 input double; U1 output double; F_prop4 input double; U2 output double; U3 output double; U4 output double; l_boom input double; anv_total output double
function [U1, U2, U3, U4, anv_total] = input(anv_prop1,F_prop1,anv_prop2,...
    F_prop2,anv_prop3,F_prop3,anv_prop4,F_prop4,l_boom)
%#eml

% Calculating Thrust in z-axis with respect to body fixed coordinate system
U1 = F_prop1 + F_prop2 + F_prop3 + F_prop4;             % [N]

% Calculating Torque around x-axis (Roll) due to Thrust
U2 = l_boom*(-F_prop4+F_prop2);                         % [Nm]

% Calculating Torque around y-axis (Pitch) due to Thrust
U3 = l_boom*(-F_prop1+F_prop3);                         % [Nm]

% Calculating Torque around z-axis (Yaw) due to Thrust
U4 = l_boom*(F_prop1-F_prop2+F_prop3-F_prop4);          % [Nm]

% Overall propeller speed
anv_total = anv_prop1-anv_prop2+anv_prop3-anv_prop4;    % [rad/s]

== matlab function Quadrocopter controller/inverted Movement Matrix ==
  data: U1 input double; F_prop1 output double; F_prop2 output double; F_prop3 output double; F_prop4 output double; U2 input double; U3 input double; U4 input double; l_boom input double
function [F_prop1,F_prop2,F_prop3,F_prop4] = fcn(U1,U2,U3,U4,l_boom)
%#eml

% Force needed at the front propeller in [N]
F_prop1 = (U1/4)-(U3/(2*l_boom))+(U4/(4*l_boom));

% Force needed at the left propeller in [N]
F_prop2 = (U1/4)+(U2/(2*l_boom))-(U4/(4*l_boom));

% Force needed at the back propeller in [N]
F_prop3 = (U1/4)+(U3/(2*l_boom))+(U4/(4*l_boom));

% Force needed at the right propeller in [N]
F_prop4 = (U1/4)-(U2/(2*l_boom))-(U4/(4*l_boom));

== matlab function Quadrocopter model/Rotation matrix ==
  data: phi input double; theta input double; psi input double; R1_1 output double; R2_1 output double; R3_1 output double; R1_2 output double; R2_2 output double; R3_2 output double; R1_3 output double; R2_3 output double; R3_3 output double
function [ R1_1, R2_1, R3_1, R1_2, R2_2, R3_2, R1_3, R2_3, R3_3] = input...
                                                    (phi, theta, psi)
% Transformation of E-frame to B-Frame
R1_1 = cos(psi)*cos(theta);
R2_1 = sin(psi)*cos(theta);
R3_1 = -sin(theta);
R1_2 = -sin(psi)*cos(phi)+cos(psi)*sin(theta)*sin(phi);
R2_2 = cos(psi)*cos(phi)+sin(psi)*sin(theta)*sin(phi);
R3_2 = cos(theta)*sin(phi);
R1_3 = sin(psi)*sin(phi)+cos(psi)*sin(theta)*cos(phi);
R2_3 = -cos(psi)*sin(phi)+sin(psi)*sin(theta)*cos(phi);
R3_3 = cos(theta)*cos(phi);
